simulink model "BMS_Template"  (R2019b)
settings: Solver=FixedStepDiscrete  StartTime=0.0  StopTime=40000  FixedStep=ts  RelTol=1e-3  EnableMultiTasking=on
InitFcn:
  | I_cc = 15;
  | V_top = 12.6;
  | V_th=11.5;
  | T_volt = 600;
  | 
  | R_bleed = 5;
  | R = 0.2;
  | numCells = 3;
  | idx = 3;
  | h_conv_end = 10;
  | h_conv = 5;
  | deltaV = 0.05;
  | cell_width = 0.2150;
  | cell_colume = 3.9732e-4;
  | cell_area = 0.1019;
  | Capacity = [31,31,31];
  | 
  | ts = 1e-1;
libraries: fl_lib x7
settings Model: Creator=mluethy  LastModifiedBy=cpatel
settings SolverCC: ConcurrentTasks=on  AutoInsertRateTranBlk=on  InsertRTBMode=Never (minimum delay)
settings DataIOCC: ExternalInput=Battery  SaveFormat=StructureWithTime  SaveState=on  SignalLoggingName=logsOut
settings OptimizationCC: BlockReduction=off  BooleanDataType=off  OptimizeBlockIOStorage=off  BufferReuse=off  GlobalBufferReuse=off  ExpressionFolding=off  LocalBlockOutputs=off  InitFltsAndDblsToZero=on  OptimizeDataStoreBuffers=off  BusAssignmentInplaceUpdate=off
settings DebuggingCC: SaveWithParameterizedLinksMsg=none  UnderspecifiedInitializationDetection=Classic  MergeDetectMultiDrivingBlocksExec=none  CheckExecutionContextPreStartOutputMsg=on  CheckExecutionContextRuntimeOutputMsg=on  SignalResolutionControl=TryResolveAllWithWarning  SFUnexpectedBacktrackingDiag=warning  SFNoUnconditionalDefaultTransitionDiag=warning  SFExecutionAtInitializationDiag=none  ArithmeticOperatorsInVariantConditions=warning
settings HardwareCC: ProdBitPerPointer=32  ProdBitPerSizeT=32  ProdBitPerPtrDiffT=32  ProdLargestAtomicFloat=None  ProdWordSize=32  ProdLongLongMode=on  ProdHWDeviceType=Generic->32-bit x86 compatible
settings ModelReferenceCC: PropagateSignalLabelsOutOfModel=off
settings SFSimCC: SimUseLocalCustomCode=off  CustomCodeUndefinedFunction=UseInterfaceOnly
settings RTWCC: Description=Simulink Real-Time  SystemTargetFile=slrt.tlc  TemplateMakefile=slrt_default_tmf  RTWUseLocalCustomCode=off  CodeExecutionProfiling=on  RTWCompilerOptimization=on
settings CodeAppCC: StateflowObjectComments=on
settings SimulinkRealTimeCC: SupportVariableSizeSignals=on  PreserveStateflowLocalDataDimensions=off  RL32LogTETModifier=off  RTWCAPISignals=on  xPCConcurrentTasks=on
settings ConfigComp: CovMetricSettings=dw  CovHtmlReporting=on  CovSaveCumulativeToWorkspaceVar=on  CovSaveSingleToWorkspaceVar=on  CovExternalEMLEnable=off  CovSFcnEnable=off

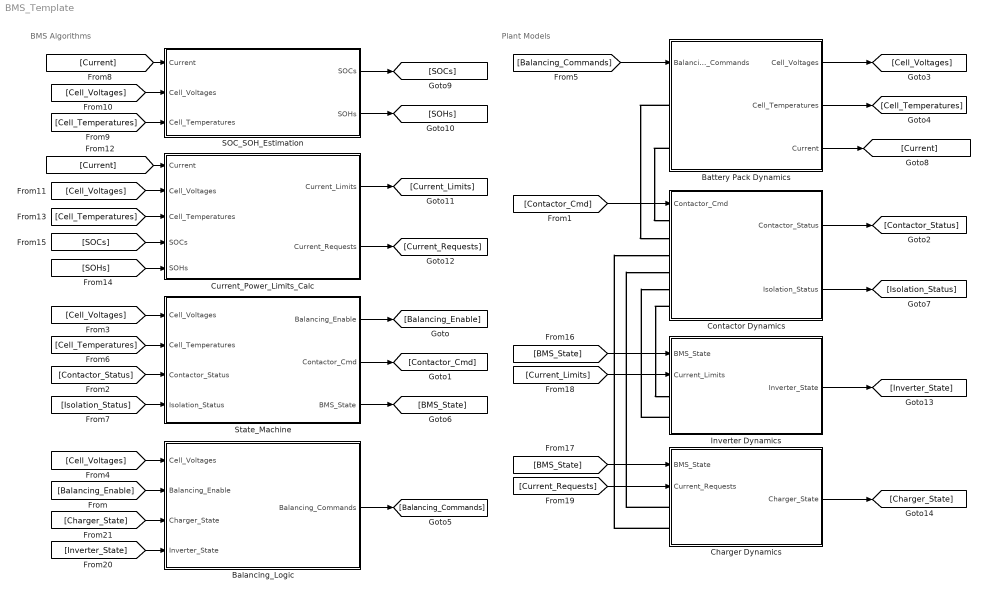
== system BMS_Template ==
  note: Plant Models
  note: BMS Algorithms
  Balancing_Logic : Subsystem
  Battery Pack Dynamics : Subsystem
  Charger Dynamics : Subsystem
  Contactor Dynamics : Subsystem
  Current_Power_Limits_Calc : Subsystem
  Inverter Dynamics : Subsystem
  SOC_SOH_Estimation : Subsystem
  State_Machine : Subsystem
  wires:
  State_Machine/1(Balancing_Enable) -> [Balancing_Enable]
  [Balancing_Enable] -> Balancing_Logic/2(Balancing_Enable)
  State_Machine/2(Contactor_Cmd) -> [Contactor_Cmd]
  [Contactor_Cmd] -> Contactor Dynamics/1(Contactor_Cmd)
  Contactor Dynamics/1(Contactor_Status) -> [Contactor_Status]
  [Contactor_Status] -> State_Machine/3(Contactor_Status)
  [Cell_Voltages] -> State_Machine/1(Cell_Voltages)
  Battery Pack Dynamics/1(Cell_Voltages) -> [Cell_Voltages]
  Battery Pack Dynamics/2(Cell_Temperatures) -> [Cell_Temperatures]
  [Cell_Voltages] -> Balancing_Logic/1(Cell_Voltages)
  Balancing_Logic/1(Balancing_Commands) -> [Balancing_Commands]
  [Balancing_Commands] -> Battery Pack Dynamics/1(Balancing_Commands)
  [Cell_Temperatures] -> State_Machine/2(Cell_Temperatures)
  State_Machine/3(BMS_State) -> [BMS_State]
  [Isolation_Status] -> State_Machine/4(Isolation_Status)
  Contactor Dynamics/2(Isolation_Status) -> [Isolation_Status]
  Battery Pack Dynamics/3(Current) -> [Current]
  [Current] -> SOC_SOH_Estimation/1(Current)
  [Cell_Temperatures] -> SOC_SOH_Estimation/3(Cell_Temperatures)
  [Cell_Voltages] -> SOC_SOH_Estimation/2(Cell_Voltages)
  SOC_SOH_Estimation/1(SOCs) -> [SOCs]
  SOC_SOH_Estimation/2(SOHs) -> [SOHs]
  [Cell_Voltages] -> Current_Power_Limits_Calc/2(Cell_Voltages)
  [Cell_Temperatures] -> Current_Power_Limits_Calc/3(Cell_Temperatures)
  [Current] -> Current_Power_Limits_Calc/1(Current)
  [SOHs] -> Current_Power_Limits_Calc/5(SOHs)
  [SOCs] -> Current_Power_Limits_Calc/4(SOCs)
  [BMS_State] -> Inverter Dynamics/1(BMS_State)
  [BMS_State] -> Charger Dynamics/1(BMS_State)
  Current_Power_Limits_Calc/1(Current_Limits) -> [Current_Limits]
  Current_Power_Limits_Calc/2(Current_Requests) -> [Current_Requests]
  [Current_Limits] -> Inverter Dynamics/2(Current_Limits)
  [Current_Requests] -> Charger Dynamics/2(Current_Requests)
  Inverter Dynamics/1(Inverter_State) -> [Inverter_State]
  Charger Dynamics/1(Charger_State) -> [Charger_State]
  [Inverter_State] -> Balancing_Logic/4(Inverter_State)
  [Charger_State] -> Balancing_Logic/3(Charger_State)
  connections:
  Inverter Dynamics/LConn2 -- Contactor Dynamics/LConn5
  Contactor Dynamics/LConn6 -- Inverter Dynamics/LConn1
  Charger Dynamics/LConn1 -- Contactor Dynamics/LConn4
  Charger Dynamics/LConn2 -- Contactor Dynamics/LConn3
  Battery Pack Dynamics/LConn1 -- Contactor Dynamics/LConn2
  Battery Pack Dynamics/LConn2 -- Contactor Dynamics/LConn1

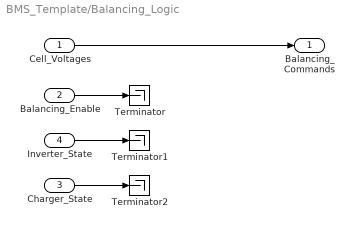
== system BMS_Template/Balancing_Logic ==
  Cell_Voltages : Inport
  Balancing_Enable : Inport  Port=2
  Charger_State : Inport  Port=3
  Inverter_State : Inport  Port=4
  Terminator : Terminator
  Terminator1 : Terminator
  Terminator2 : Terminator
  Balancing_Commands : Outport  VectorParamsAs1DForOutWhenUnconnected=off
  wires:
  Cell_Voltages/1 -> Balancing_Commands/1
  Balancing_Enable/1 -> Terminator/1
  Inverter_State/1 -> Terminator1/1
  Charger_State/1 -> Terminator2/1

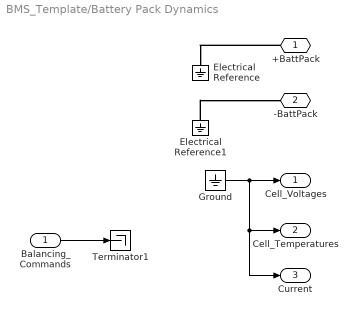
== system BMS_Template/Battery Pack Dynamics ==
  Balancing_Commands : Inport
  Electrical Reference : fl_lib/Electrical/Electrical Elements/Electrical Reference
  Electrical Reference1 : fl_lib/Electrical/Electrical Elements/Electrical Reference
  Ground : Ground
  Terminator1 : Terminator
  +BattPack : PMIOPort  Side=Left
  -BattPack : PMIOPort  Port=2  Side=Left
  Cell_Voltages : Outport  VectorParamsAs1DForOutWhenUnconnected=off
  Cell_Temperatures : Outport  Port=2  VectorParamsAs1DForOutWhenUnconnected=off
  Current : Outport  Port=3  VectorParamsAs1DForOutWhenUnconnected=off
  wires:
  Ground/1 -> Cell_Temperatures/1, Current/1, Cell_Voltages/1
  Balancing_Commands/1 -> Terminator1/1
  connections:
  +BattPack/RConn1 -- Electrical Reference/LConn1
  Electrical Reference1/LConn1 -- -BattPack/RConn1

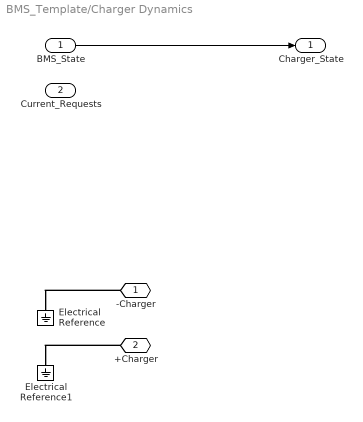
== system BMS_Template/Charger Dynamics ==
  BMS_State : Inport
  Current_Requests : Inport  Port=2
  Electrical Reference : fl_lib/Electrical/Electrical Elements/Electrical Reference
  Electrical Reference1 : fl_lib/Electrical/Electrical Elements/Electrical Reference
  -Charger : PMIOPort  Side=Left
  +Charger : PMIOPort  Port=2  Side=Left
  Charger_State : Outport  VectorParamsAs1DForOutWhenUnconnected=off
  wires:
  BMS_State/1 -> Charger_State/1
  connections:
  +Charger/RConn1 -- Electrical Reference1/LConn1
  -Charger/RConn1 -- Electrical Reference/LConn1

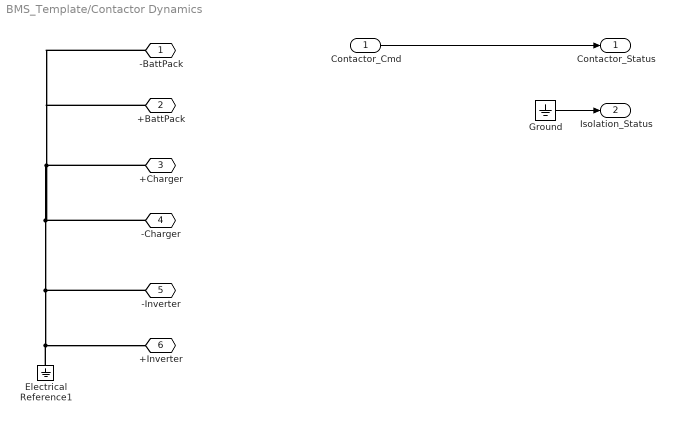
== system BMS_Template/Contactor Dynamics ==
  Contactor_Cmd : Inport
  Electrical Reference1 : fl_lib/Electrical/Electrical Elements/Electrical Reference
  Ground : Ground
  -BattPack : PMIOPort  Side=Left
  +BattPack : PMIOPort  Port=2  Side=Left
  +Charger : PMIOPort  Port=3  Side=Left
  -Charger : PMIOPort  Port=4  Side=Left
  -Inverter : PMIOPort  Port=5  Side=Left
  +Inverter : PMIOPort  Port=6  Side=Left
  Contactor_Status : Outport  VectorParamsAs1DForOutWhenUnconnected=off
  Isolation_Status : Outport  Port=2  VectorParamsAs1DForOutWhenUnconnected=off
  wires:
  Contactor_Cmd/1 -> Contactor_Status/1
  Ground/1 -> Isolation_Status/1
  connections:
  Electrical Reference1/LConn1 -- -BattPack/RConn1 -- +BattPack/RConn1 -- +Charger/RConn1 -- -Charger/RConn1 -- -Inverter/RConn1 -- +Inverter/RConn1

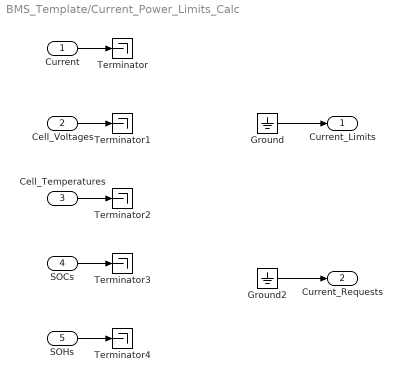
== system BMS_Template/Current_Power_Limits_Calc ==
  Current : Inport
  Cell_Voltages : Inport  Port=2
  Cell_Temperatures : Inport  Port=3
  SOCs : Inport  Port=4
  SOHs : Inport  Port=5
  Ground : Ground
  Ground2 : Ground
  Terminator{,1..4} (5 alike) : Terminator
  Current_Limits : Outport  VectorParamsAs1DForOutWhenUnconnected=off
  Current_Requests : Outport  Port=2  VectorParamsAs1DForOutWhenUnconnected=off
  wires:
  Current/1 -> Terminator/1
  Cell_Temperatures/1 -> Terminator2/1
  Cell_Voltages/1 -> Terminator1/1
  SOCs/1 -> Terminator3/1
  SOHs/1 -> Terminator4/1
  Ground2/1 -> Current_Requests/1
  Ground/1 -> Current_Limits/1

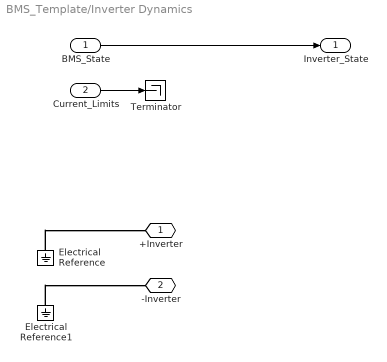
== system BMS_Template/Inverter Dynamics ==
  BMS_State : Inport
  Current_Limits : Inport  Port=2
  Electrical Reference : fl_lib/Electrical/Electrical Elements/Electrical Reference
  Electrical Reference1 : fl_lib/Electrical/Electrical Elements/Electrical Reference
  Terminator : Terminator
  +Inverter : PMIOPort  Side=Left
  -Inverter : PMIOPort  Port=2  Side=Left
  Inverter_State : Outport  VectorParamsAs1DForOutWhenUnconnected=off
  wires:
  BMS_State/1 -> Inverter_State/1
  Current_Limits/1 -> Terminator/1
  connections:
  Electrical Reference1/LConn1 -- -Inverter/RConn1
  Electrical Reference/LConn1 -- +Inverter/RConn1

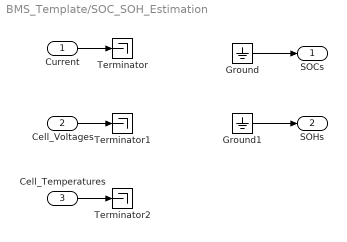
== system BMS_Template/SOC_SOH_Estimation ==
  Current : Inport
  Cell_Voltages : Inport  Port=2
  Cell_Temperatures : Inport  Port=3
  Ground : Ground
  Ground1 : Ground
  Terminator : Terminator
  Terminator1 : Terminator
  Terminator2 : Terminator
  SOCs : Outport  VectorParamsAs1DForOutWhenUnconnected=off
  SOHs : Outport  Port=2  VectorParamsAs1DForOutWhenUnconnected=off
  wires:
  Current/1 -> Terminator/1
  Cell_Voltages/1 -> Terminator1/1
  Cell_Temperatures/1 -> Terminator2/1
  Ground/1 -> SOCs/1
  Ground1/1 -> SOHs/1

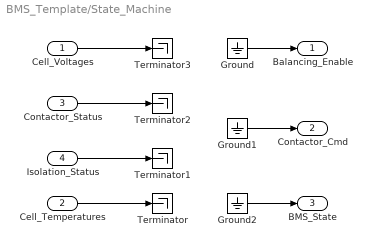
== system BMS_Template/State_Machine ==
  Cell_Voltages : Inport
  Cell_Temperatures : Inport  Port=2
  Contactor_Status : Inport  Port=3
  Isolation_Status : Inport  Port=4
  Ground : Ground
  Ground1 : Ground
  Ground2 : Ground
  Terminator{,1..3} (4 alike) : Terminator
  Balancing_Enable : Outport  VectorParamsAs1DForOutWhenUnconnected=off
  Contactor_Cmd : Outport  Port=2  VectorParamsAs1DForOutWhenUnconnected=off
  BMS_State : Outport  Port=3  VectorParamsAs1DForOutWhenUnconnected=off
  wires:
  Ground/1 -> Balancing_Enable/1
  Ground1/1 -> Contactor_Cmd/1
  Ground2/1 -> BMS_State/1
  Cell_Temperatures/1 -> Terminator/1
  Isolation_Status/1 -> Terminator1/1
  Contactor_Status/1 -> Terminator2/1
  Cell_Voltages/1 -> Terminator3/1
